simulink model "sule_tunc6"  (Simulink 8.4)
settings: Solver=ode23tb  StartTime=0.0  StopTime=3  RelTol=1e-3
undefined symbols (not defined in the file): sigbuilder_block
libraries: powerlib x18, powerlib_meascontrol x2
settings Model: Creator=asus1  LastModifiedBy=asus1
settings DataIOCC: SignalLoggingSaveFormat=Dataset
settings OptimizationCC: ExpressionDepthLimit=128
settings DebuggingCC: UnderspecifiedInitializationDetection=Simplified  MergeDetectMultiDrivingBlocksExec=error  FcnCallInpInsideContextMsg=EnableAllAsError  StateNameClashWarn=none
settings GRTTargetCC: CombineOutputUpdateFcns=on  GRTInterface=off

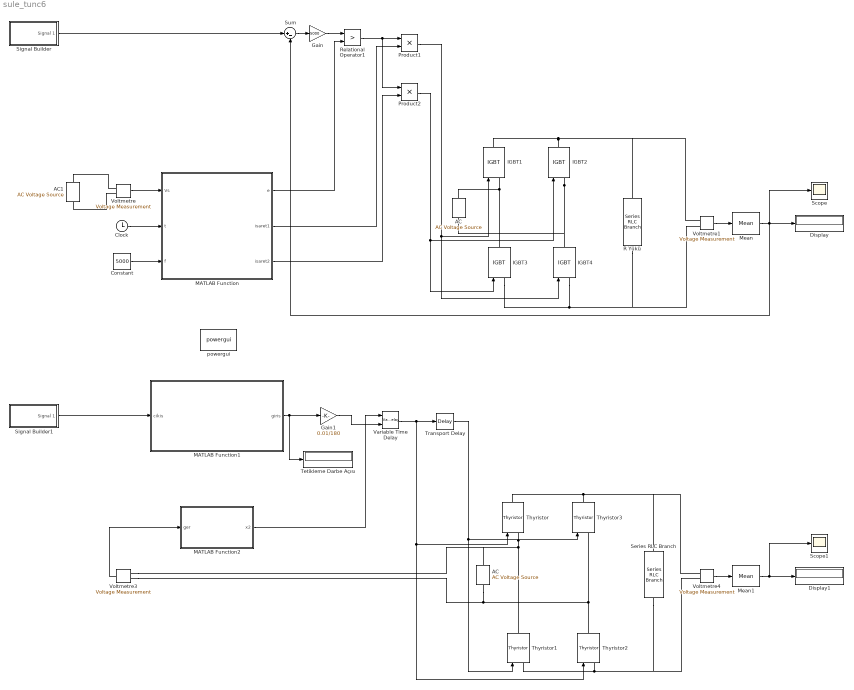
== system sule_tunc6 ==
  AC : powerlib/Electrical Sources/AC Voltage Source  Amplitude=220*sqrt(2)  Phase=0  Frequency=50  SampleTime=0  Measurements=None
  "AC " : powerlib/Electrical Sources/AC Voltage Source  Amplitude=220*sqrt(2)  Phase=0  Frequency=50  SampleTime=0  Measurements=None
  AC1 : powerlib/Electrical Sources/AC Voltage Source  Amplitude=220*sqrt(2)  Phase=0  Frequency=50  SampleTime=0  Measurements=None
  Clock : Clock
  Constant : Constant  Value=5000
  Display : Display
  Display1 : Display
  Gain : Gain  Gain=5000
  Gain1 : Gain  Gain=0.01/180
  IGBT{1..4} (4 alike) : powerlib/Power Electronics/IGBT  Ron=0.001  Lon=0  Vf=0.001  Tf=1e-6  Tt=2e-6  IC=0  Rs=1e5  Cs=inf  Measurements=off
  MATLAB Function : MATLAB Function  TreatAsAtomicUnit=on
  MATLAB Function1 : MATLAB Function  TreatAsAtomicUnit=on
  MATLAB Function2 : MATLAB Function  TreatAsAtomicUnit=on
  Mean : powerlib_meascontrol/Measurements/Mean  Freq=50  Vinit=0  Ts=0
  Mean1 : powerlib_meascontrol/Measurements/Mean  Freq=50  Vinit=0  Ts=0
  Product1 : Product
  Product2 : Product
  R Yükü : powerlib/Elements/Series RLC Branch  LConnTagsString=__new0  RConnTagsString=__new0  BranchType=R  Resistance=10  Inductance=1e-3  SetiL0=off  InitialCurrent=0  Capacitance=1e-6  Setx0=off  InitialVoltage=0  Measurements=None
  Relational Operator1 : RelationalOperator  Operator=>  OutDataTypeStr=boolean
  Scope : Scope
      settings: TimeRange=3  YMin=0  YMax=200
  Scope1 : Scope
      settings: TimeRange=3  YMin=0  YMax=200
  Series RLC Branch : powerlib/Elements/Series RLC Branch  LConnTagsString=__new0  RConnTagsString=__new0  BranchType=R  Resistance=10  Inductance=1e-3  SetiL0=off  InitialCurrent=0  Capacitance=1e-6  Setx0=off  InitialVoltage=0  Measurements=None
  Signal Builder : Subsystem  Tag=STV Subsys  LoadFcn=sigbuilder_block('load');  StartFcn=sigbuilder_block('start');  StopFcn=sigbuilder_block('stop');  ClipboardFcn=sigbuilder_block('clipboard');  mask(Sigbuilder block){}
      mask help: Simulink:masks:SigbuilderBlock_MD
      mask init:
      | if ~strcmp(get_param(bdroot(gcbh),'SimulationStatus'),'stopped') tuvar = sigbuilder_block('maskInit'); end
      settings: CopyFcn=sigbuilder_block('copy');  DeleteFcn=sigbuilder_block('delete');  ModelCloseFcn=sigbuilder_block('modelClose');  PreSaveFcn=sigbuilder_block('preSave');  PauseFcn=sigbuilder_block('pause');  ContinueFcn=sigbuilder_block('continue');  NameChangeFcn=sigbuilder_block('namechange');  OpenFcn=sigbuilder_block('open',[437.6 199.2 550.4 400 ]);  CloseFcn=sigbuilder_block('close');
      mask Display: plot(0, 0, 100, 100,[2, 2, 32, 32, 2], [68, 8, 8, 68, 68],[32, 2], [38, 38], [32, 19, 2],[53, 60, 44], [32, 17, 17, 2],[16, 16, 31, 31]);txt = getActiveGroup(gcbh);text(2, 100, txt,'verticalAlignment', 'top');
  Signal Builder1 : Subsystem  Tag=STV Subsys  LoadFcn=sigbuilder_block('load');  StartFcn=sigbuilder_block('start');  StopFcn=sigbuilder_block('stop');  ClipboardFcn=sigbuilder_block('clipboard');  mask(Sigbuilder block){}
      mask help: Simulink:masks:SigbuilderBlock_MD
      mask init:
      | if ~strcmp(get_param(bdroot(gcbh),'SimulationStatus'),'stopped') tuvar = sigbuilder_block('maskInit'); end
      settings: CopyFcn=sigbuilder_block('copy');  DeleteFcn=sigbuilder_block('delete');  ModelCloseFcn=sigbuilder_block('modelClose');  PreSaveFcn=sigbuilder_block('preSave');  PauseFcn=sigbuilder_block('pause');  ContinueFcn=sigbuilder_block('continue');  NameChangeFcn=sigbuilder_block('namechange');  OpenFcn=sigbuilder_block('open',[437.6 199.2 550.4 400 ]);  CloseFcn=sigbuilder_block('close');
      mask Display: plot(0, 0, 100, 100,[2, 2, 32, 32, 2], [68, 8, 8, 68, 68],[32, 2], [38, 38], [32, 19, 2],[53, 60, 44], [32, 17, 17, 2],[16, 16, 31, 31]);txt = getActiveGroup(gcbh);text(2, 100, txt,'verticalAlignment', 'top');
  Sum : Sum  Inputs=|+-
  Tetikleme Darbe Açısı : Display
  Thyristor{,1..3} (4 alike) : powerlib/Power Electronics/Thyristor  Ron=0.001  Lon=0  Vf=0.001  IC=0  Rs=1e5  Cs=inf  Measurements=off
  Transport Delay : TransportDelay  DelayTime=0.01
  Variable Time Delay : VariableTransportDelay  MaximumDelay=10
  Voltmetre{,1,3..4} (4 alike) : powerlib/Measurements/Voltage Measurement  PhasorSimulation=off  OutputType=Complex  PSBequivalent=0
  powergui : powerlib/powergui  Priority=1  SimulationMode=Discrete  SolverType=Tustin  SampleTime=1e-6  frequency=60  SPID=off  DisableSnubberDevices=off  DisableRonSwitches=off  DisableVfSwitches=off  SwTol=0  DisplayEquations=off  Interpol=off  methode=off  Ts=100  frequencyindice=50  Pbase=100e6  ErrMax=1e-4  Iterations=50  UnitsV=kV  UnitsW=MW  FunctionMessages=off  echomessages=off  HookPort=off  EnableUseOfTLC=off  x0status=blocks  RestoreLinks=warning  ResistiveCurrentMeasurement=off  Frange=[0:2:500]  Ylog=off  Xlog=on  ShowGrid=off  save=off  variable=ZData  structure=0  ZoomFFT=off  StartTime=0.0  cycles=1  DisplayStyle=1  fundamental=60  FreqAxis=off  MaxFrequency=1000  frequencyindicesteady=1  RmsSteady=1  display=off
  wires:
  Voltmetre/1 -> MATLAB Function/1(Vs)
  Clock/1 -> MATLAB Function/2(t)
  Constant/1 -> MATLAB Function/3(f)
  Voltmetre1/1 -> Mean/1
  Signal Builder/1(Signal 1) -> Sum/1
  Sum/1 -> Gain/1
  MATLAB Function/1(e) -> Relational Operator1/2
  Gain/1 -> Relational Operator1/1
  Relational Operator1/1 -> Product1/1, Product2/1
  MATLAB Function/2(isaret1) -> Product1/2
  MATLAB Function/3(isaret2) -> Product2/2
  Product1/1 -> IGBT1/1, IGBT4/1
  Product2/1 -> IGBT2/1, IGBT3/1
  Mean/1 -> Display/1, Sum/2, Scope/1
  Transport Delay/1 -> Thyristor3/1, Thyristor1/1
  Variable Time Delay/1 -> Transport Delay/1, Thyristor/1, Thyristor2/1
  Voltmetre4/1 -> Mean1/1
  Mean1/1 -> Display1/1, Scope1/1
  Signal Builder1/1(Signal 1) -> MATLAB Function1/1(cikis)
  MATLAB Function1/1(giris) -> Gain1/1, Tetikleme Darbe Açısı/1
  Voltmetre3/1 -> MATLAB Function2/1(ger)
  MATLAB Function2/1(x2) -> Variable Time Delay/1
  Gain1/1 -> Variable Time Delay/2
  connections:
  IGBT2/LConn1 -- IGBT4/RConn1 -- "AC "/LConn1
  "AC "/RConn1 -- IGBT1/LConn1 -- IGBT3/RConn1
  IGBT2/RConn1 -- IGBT1/RConn1 -- R Yükü/LConn1 -- Voltmetre1/LConn1
  IGBT4/LConn1 -- IGBT3/LConn1 -- R Yükü/RConn1 -- Voltmetre1/LConn2
  AC/LConn1 -- Voltmetre3/LConn2 -- Thyristor2/RConn1 -- Thyristor3/LConn1
  Thyristor/LConn1 -- Thyristor1/RConn1 -- AC/RConn1 -- Voltmetre3/LConn1
  Thyristor3/RConn1 -- Thyristor/RConn1 -- Voltmetre4/LConn1 -- Series RLC Branch/LConn1
  Thyristor2/LConn1 -- Thyristor1/LConn1 -- Voltmetre4/LConn2 -- Series RLC Branch/RConn1
  Voltmetre/LConn1 -- AC1/RConn1
  Voltmetre/LConn2 -- AC1/LConn1

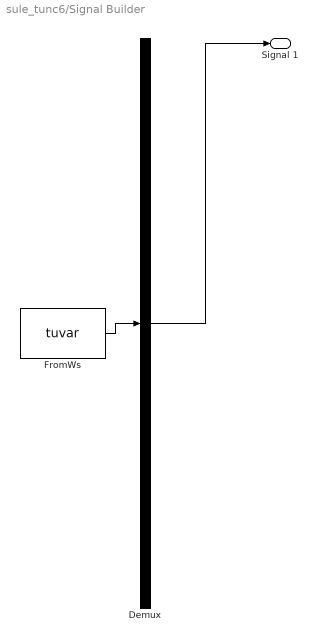
== system sule_tunc6/Signal Builder ==
  Demux : Demux  Tag=STV Demux  Outputs=1
  FromWs : FromWorkspace  Tag=STV FromWs  VariableName=tuvar  SampleTime=0  SigBuilderData=DataTag0  VnvData=DataTag1
      SigBuilderData=|
      | common.afterFinalStr = 'Extrapolate'
      | common.sampleTime = 0
      | dataSet.timeRange = [0 10]
      | dataSet.name = 'Group 1'
      | sbobj.Groups.Name = 'Group 1'
      | sbobj.Groups.Signals.Name = 'Signal 1'
      | sbobj.Groups.Signals.XData = [0 0.5 0.5 1 1 1.5 1.5 2 2 2.5 2.5 4 4 6 6 10]
      | sbobj.Groups.Signals.YData = [180 180 140 140 100 100 60 60 20 20 10 10 1 1 0 0]
  Signal 1 : Outport  Tag=STV Outport
  wires:
  Demux/1 -> Signal 1/1
  FromWs/1 -> Demux/1

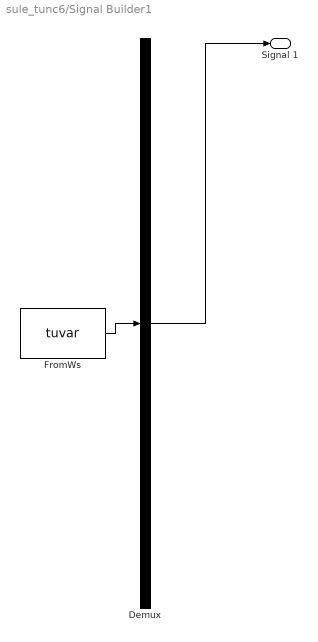
== system sule_tunc6/Signal Builder1 ==
  Demux : Demux  Tag=STV Demux  Outputs=1
  FromWs : FromWorkspace  Tag=STV FromWs  VariableName=tuvar  SampleTime=0  SigBuilderData=DataTag2  VnvData=DataTag3
      SigBuilderData=|
      | common.afterFinalStr = 'Extrapolate'
      | common.sampleTime = 0
      | dataSet.timeRange = [0 10]
      | dataSet.name = 'Group 1'
      | sbobj.Groups.Name = 'Group 1'
      | sbobj.Groups.Signals.Name = 'Signal 1'
      | sbobj.Groups.Signals.XData = [0 0.5 0.5 1 1 1.5 1.5 2 2 2.5 2.5 4 4 6 6 10]
      | sbobj.Groups.Signals.YData = [180 180 140 140 100 100 60 60 20 20 10 10 1 1 0 0]
  Signal 1 : Outport  Tag=STV Outport
  wires:
  Demux/1 -> Signal 1/1
  FromWs/1 -> Demux/1

== matlab function MATLAB Function1 ==
  data: cikis input double; giris output double
function giris=istenen(cikis)
fi=2;
e=0.00001; 
max=20; 
fark=0.000001; 
giris=0;
f=0;
V=220*sqrt(2); 
for k=1:max
    b=(V/pi)*sin(fi); 
    giris=fi-(-(V/pi)*(cos(fi)+1)+cikis)/b;  
    u=abs(giris-fi);
    u1=2*u/(abs(giris)+fark);
    fi=giris;
    f=(-(V/pi)*(cos(fi)+1)+cikis);
if (u<fark)||(u1<fark)||(abs(f)<e);
    break
end 
end
giris=giris*180/pi;

== matlab function MATLAB Function ==
  data: Vs input double; e output double; t input double; f input double; isaret1 output double; isaret2 output double
function [e,isaret1,isaret2] = periyodik(Vs,t,f)
% bu programda ucgen dalga T/2 icinde d.c isaret bicimindedir.
isaret1=0;
isaret2=0;
T=1/f;
V=1;
m=2*f*V;
e=0;
b=fix(t/T);
   if (t>=b*T) && t<=(b+0.5)*T
       e=m*(t-(b+0.5)*T)+V;
   end
   if ( t>(0.5+b)*T && t<=(b+1)*T)
       e=-m*(t-(b+0.5)*T)+V;
   end
   e=abs(e);
   if Vs>0
       isaret1=1;
       isaret2=0;
   else
       isaret1=0;
       isaret2=1;
   end

== matlab function MATLAB Function2 ==
  data: x2 output double; ger input double
function x2=fcn1(ger)
R=10;
epsilon=0.000001;
if ger>0
    x2=1;
else
    x2=0;
end
